simulink model "TDDO_sim"  (Simulink 8.8)
settings: Solver=VariableStepAuto  StartTime=0.0  StopTime=100.0  RelTol=1e-3
settings Model: SuppressorTable=22 serialization::archive 11 0 3 0 0 0 0 0  Creator=guoshaopan  LastModifiedBy=guoshaopan
settings DataIOCC: LimitDataPoints=off  SaveFormat=Dataset  SignalLoggingSaveFormat=Dataset
settings OptimizationCC: LifeSpan=auto
settings DebuggingCC: UnderspecifiedInitializationDetection=Simplified  MergeDetectMultiDrivingBlocksExec=error  FcnCallInpInsideContextMsg=error  StateNameClashWarn=none  SFUnexpectedBacktrackingDiag=error  SFNoUnconditionalDefaultTransitionDiag=error  SFExecutionAtInitializationDiag=warning
settings HardwareCC: ProdBitPerPointer=64  ProdBitPerSizeT=64  ProdBitPerPtrDiffT=64  ProdLargestAtomicFloat=Float  ProdIntDivRoundTo=Zero  ProdEndianess=LittleEndian  ProdWordSize=64  ProdHWDeviceType=Intel->x86-64 (Windows64)
settings ModelReferenceCC: PropagateSignalLabelsOutOfModel=on
settings GRTTargetCC: TargetLangStandard=C99 (ISO)  GeneratePreprocessorConditionals=Use local settings  CombineOutputUpdateFcns=on  GRTInterface=off
settings ConfigComp: CovMetricSettings=dwe  CovHtmlReporting=off  CovSaveCumulativeToWorkspaceVar=off  CovSaveSingleToWorkspaceVar=off  CovExternalEMLEnable=on

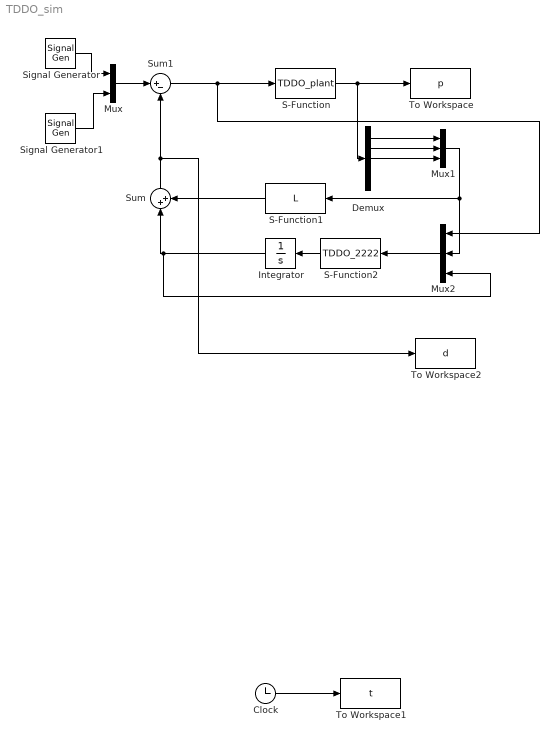
== system TDDO_sim ==
  Clock : Clock
  Demux : Demux  Outputs=5
  Integrator : Integrator
  Mux : Mux  Inputs=2
  Mux1 : Mux  Inputs=3
  Mux2 : Mux  Inputs=3
  S-Function : S-Function  FunctionName=TDDO_plant  SFunctionDeploymentMode=off  EnableBusSupport=off
  S-Function1 : S-Function  FunctionName=L  SFunctionDeploymentMode=off  EnableBusSupport=off
  S-Function2 : S-Function  FunctionName=TDDO_2222  SFunctionDeploymentMode=off  EnableBusSupport=off
  Signal Generator : SignalGenerator  Units=rad/sec
  Signal Generator1 : SignalGenerator  Amplitude=8  Units=rad/sec
  Sum : Sum  Inputs=|++
  Sum1 : Sum  Inputs=|+-
  To Workspace : ToWorkspace  VariableName=p  SampleTime=-1
  To Workspace1 : ToWorkspace  VariableName=t  SampleTime=-1
  To Workspace2 : ToWorkspace  VariableName=d  SampleTime=-1
  wires:
  Signal Generator/1 -> Mux/1
  Signal Generator1/1 -> Mux/2
  S-Function/1 -> Demux/1, To Workspace/1
  Clock/1 -> To Workspace1/1
  Mux1/1 -> Mux2/2, S-Function1/1
  S-Function1/1 -> Sum/2
  Mux/1 -> Sum1/1
  Sum/1 -> To Workspace2/1, Sum1/2
  Sum1/1 -> Mux2/1, S-Function/1
  Mux2/1 -> S-Function2/1
  Demux/1 -> Mux1/1
  Demux/2 -> Mux1/2
  Demux/3 -> Mux1/3
  S-Function2/1 -> Integrator/1
  Integrator/1 -> Mux2/3, Sum/1
